simulink model "Lista5"  (R2023a)
settings: Solver=VariableStepAuto  StartTime=0.0  StopTime=10.0  RelTol=1e-3
libraries: fl_lib x5, nesl_utility x3, sdl_lib x1
settings Model: Creator=gutoc  LastModifiedBy=gutoc

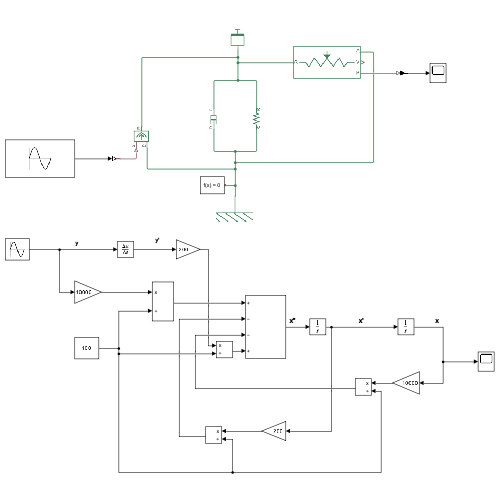
[thumbnail: Simulink's stored preview of the top-level diagram]
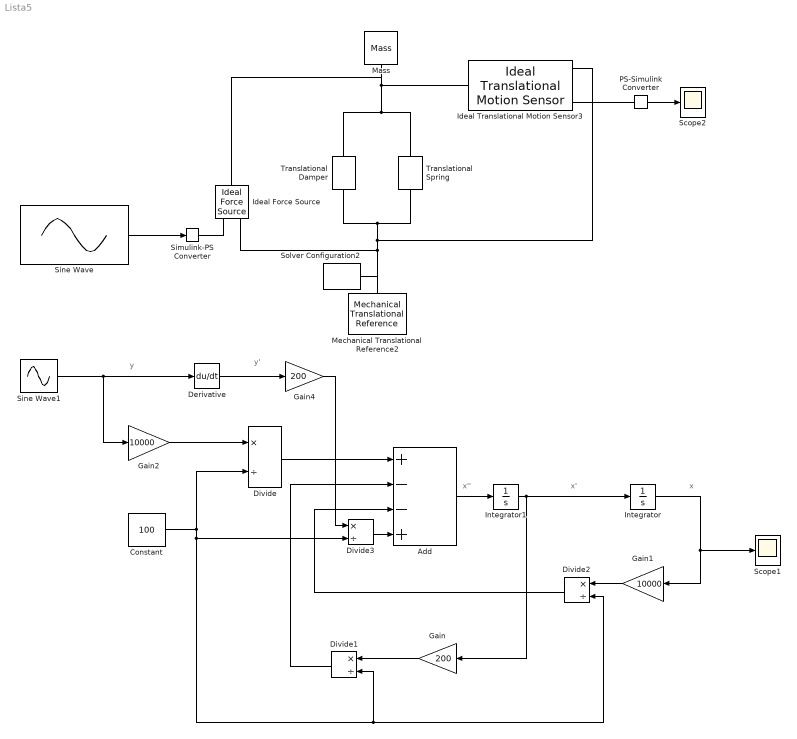
== system Lista5 ==
  note: x''
  note: y
  note: y'
  note: x'
  note: x
  Add : Sum  Inputs=+--+
  Constant : Constant  Value=100
  Derivative : Derivative
  Divide{,1..3} (4 alike) : Product  Inputs=*/
  Gain : Gain  Gain=200
  Gain1 : Gain  Gain=10000
  Gain2 : Gain  Gain=10000
  Gain4 : Gain  Gain=200
  Ideal Force Source : fl_lib/Mechanical/Mechanical Sources/Ideal Force Source
  Ideal Translational Motion Sensor3 : fl_lib/Mechanical/Mechanical Sensors/Ideal Translational Motion Sensor  reference=foundation.enum.MeasurementReference.difference  acceleration_port=false  velocity_port=true  position_port=true  offset=0 m
  Integrator : Integrator
  Integrator1 : Integrator
  Mass : fl_lib/Mechanical/Translational Elements/Mass  mass=100 kg  num_ports=foundation.enum.numPorts2.one  v_specify=off  v_priority=High  v=0 m/s  v_nominal_specify=off  v_nominal_unit=m/s  v_nominal_value=1  f_specify=off  f_priority=None  f=0 N  f_nominal_specify=off  f_nominal_unit=N  f_nominal_value=1
  Mechanical Translational Reference2 : fl_lib/Mechanical/Translational Elements/Mechanical Translational Reference
  PS-Simulink Converter : nesl_utility/PS-Simulink Converter  PhysicalDomain=network_engine_domain  SubClassName=ps_output  LeftPortType=input  RightPortType=output  PseudoPeriodic=off  Frequencies=[]  VectorFormat=inherit  Unit=inherit  AffineConversion=off
  Scope1 : Scope
  Scope2 : Scope
  Simulink-PS Converter : nesl_utility/Simulink-PS Converter  PhysicalDomain=network_engine_domain  SubClassName=ps_input  LeftPortType=input  RightPortType=output  PseudoPeriodic=off  Frequencies=[]  NoiseDistribution=none  NoiseParameters=[]  Unit=1  AffineConversion=off  FilteringAndDerivatives=provide  SimscapeFilterOrder=1  InputFilterTimeConstant=0.001  UdotUserProvided=0
  Sine Wave : Sin  Amplitude=0.1  SampleTime=0
  Sine Wave1 : Sin  Amplitude=0.1  SampleTime=0
  Solver Configuration2 : nesl_utility/Solver Configuration  PhysicalDomain=network_engine_domain  SubClassName=solver  LeftPortType=input  RightPortType=generic  Tones=[]  Harmonics=[]  SimulateNoise=off  Profile=off  UseLocalSampling=off  EnableSwitchedLinearOptims=on  FrequencyDomain=off  UseCCode=off  RelTol=0.001  AbsTol=1e-06  MinStep=1e-09  ToWorkspace=off  RevertToSquareIcSolve=off  NumHomotopyIterations=100  PhasorMode=off  PhasorModeNumHarmonics=1  ConsistencySolver=NEWTON_FTOL  IndexReductionMethod=DerivativeReplacement  DoDC=off  ResidualTolerance=1e-09  ConsistencyTolSource=GLOBAL  ConsistencyAbsTol=0.001  ConsistencyRelTol=0.001  ConsistencyTolFactor=0.001  UseLocalSolver=off  LocalSolverChoice=NE_BACKWARD_EULER_ADVANCER  ResolveIndetEquations=on  FunctionEvalNumThread=1  LocalSolverSampleTime=0.001  DoFixedCost=off  MaxNonlinIter=3  MaxModeIter=2  ComputeImpulses=off  ImpulseIterations=2  LinearAlgebra=Sparse  LinearAlgebraNumThread=0  EquationFormulation=NE_TIME_EF  DelaysMemoryBudget=1024  AutomaticFiltering=on  FilteringTimeConstant=0.001  PartitionStorageMethod=AS_NEEDED  PartitionMemoryBudget=1024  PartitionMethod=FAST
  Translational Damper : sdl_lib/Couplings & Drives/Springs & Dampers/Translational Damper  D=200 N*s/m  enable_faults=simscape.enum.onoff.off  b_fault=1e6 N*s/m  temporal_fault=simscape.enum.onoff.off  fault_time=5 s  shock_fault=simscape.enum.onoff.off  acceleration_limit=100 m/s^2  shock_limit=1  report_fault=simscape.enum.assert.action.none  thermal_port=simscape.enum.thermaleffects.omit  thermal_mass=50 kJ/K  temperature_specify=off  temperature_priority=High  temperature=300 K  temperature_nominal_specify=off  temperature_nominal_unit=K  temperature_nominal_value=1
  Translational Spring : fl_lib/Mechanical/Translational Elements/Translational Spring  spr_rate=10000 N/m  v_specify=off  v_priority=None  v=0 m/s  v_nominal_specify=off  v_nominal_unit=m/s  v_nominal_value=1  f_specify=off  f_priority=None  f=0 N  f_nominal_specify=off  f_nominal_unit=N  f_nominal_value=1  x_specify=off  x_priority=High  x=0 m  x_nominal_specify=off  x_nominal_unit=m  x_nominal_value=1
  wires:
  PS-Simulink Converter/1 -> Scope2/1
  Constant/1 -> Divide/2, Divide2/2, Divide1/2, Divide3/2
  Sine Wave1/1 -> Derivative/1, Gain2/1
  Divide/1 -> Add/1
  Add/1 -> Integrator1/1
  Integrator1/1 -> Integrator/1, Gain/1
  Integrator/1 -> Gain1/1, Scope1/1
  Gain/1 -> Divide1/1
  Divide1/1 -> Add/2
  Gain1/1 -> Divide2/1
  Divide2/1 -> Add/3
  Derivative/1 -> Gain4/1
  Gain2/1 -> Divide/1
  Gain4/1 -> Divide3/1
  Divide3/1 -> Add/4
  Sine Wave/1 -> Simulink-PS Converter/1
  connections:
  Translational Spring/RConn1 -- Mechanical Translational Reference2/LConn1 -- Solver Configuration2/RConn1 -- Ideal Force Source/RConn2 -- Ideal Translational Motion Sensor3/RConn1 -- Translational Damper/LConn1
  Simulink-PS Converter/RConn1 -- Ideal Force Source/RConn1
  Translational Damper/RConn1 -- Ideal Translational Motion Sensor3/LConn1 -- Ideal Force Source/LConn1 -- Mass/LConn1 -- Translational Spring/LConn1
  Ideal Translational Motion Sensor3/RConn3 -- PS-Simulink Converter/LConn1
